simulink model "axi_stream_template"  (R2018a)
settings: Solver=VariableStepAuto  StartTime=0.0  StopTime=300  RelTol=1e-3
libraries: xbsIndex_r4 x18, hdlsllib x5, simulink x1
settings Model: Creator=David Northcote  LastModifiedBy=David Northcote

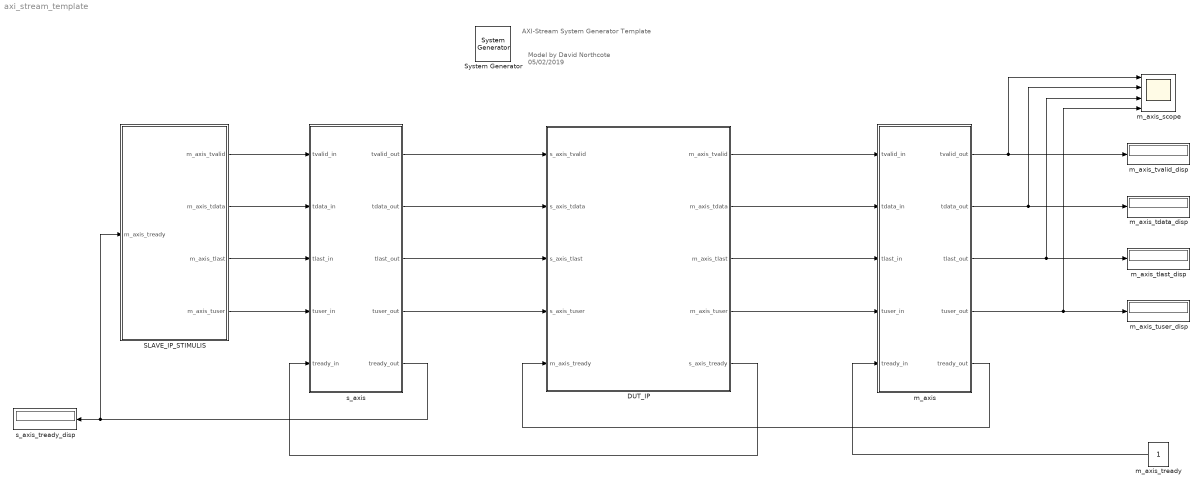
== system axi_stream_template ==
  note: Model by David Northcote
      | 05/02/2019
  note: AXI-Stream System Generator Template
  " System Generator" : xbsIndex_r4/ System Generator  Tag=genX  xilinxfamily=zynq  part=xc7z020  speed=-1  package=clg400  synthesis_tool=Vivado  clock_wrapper=Clock Enables  directory=./netlist  proj_type=Vivado  Synth_file=Vivado Synthesis Defaults  Impl_file=Vivado Implementation Defaults  testbench=off  simulink_period=1  sysclk_period=10  dcm_input_clock_period=10  incr_netlist=off  trim_vbits=Everywhere in SubSystem  dbl_ovrd=According to Block Masks  core_generation=According to Block Masks  run_coregen=off  deprecated_control=off  eval_field=0  block_type=sysgen
  DUT_IP : Subsystem
  SLAVE_IP_STIMULIS : Subsystem
  m_axis : Subsystem
  m_axis_scope : Scope  NumInputPorts=4
  m_axis_tdata_disp : Display
  m_axis_tlast_disp : Display
  m_axis_tready : Constant  VectorParams1D=off  SampleTime=-1
  m_axis_tuser_disp : Display
  m_axis_tvalid_disp : Display
  s_axis : Subsystem
  s_axis_tready_disp : Display
  wires:
  m_axis_tready/1 -> m_axis/5(tready_in)
  s_axis/5(tready_out) -> s_axis_tready_disp/1, SLAVE_IP_STIMULIS/1(m_axis_tready)
  m_axis/1(tvalid_out) -> m_axis_scope/1, m_axis_tvalid_disp/1
  m_axis/3(tlast_out) -> m_axis_scope/3, m_axis_tlast_disp/1
  m_axis/4(tuser_out) -> m_axis_scope/4, m_axis_tuser_disp/1
  m_axis/2(tdata_out) -> m_axis_scope/2, m_axis_tdata_disp/1
  s_axis/1(tvalid_out) -> DUT_IP/1(s_axis_tvalid)
  s_axis/2(tdata_out) -> DUT_IP/2(s_axis_tdata)
  s_axis/3(tlast_out) -> DUT_IP/3(s_axis_tlast)
  s_axis/4(tuser_out) -> DUT_IP/4(s_axis_tuser)
  m_axis/5(tready_out) -> DUT_IP/5(m_axis_tready)
  DUT_IP/5(s_axis_tready) -> s_axis/5(tready_in)
  DUT_IP/1(m_axis_tvalid) -> m_axis/1(tvalid_in)
  DUT_IP/2(m_axis_tdata) -> m_axis/2(tdata_in)
  DUT_IP/3(m_axis_tlast) -> m_axis/3(tlast_in)
  DUT_IP/4(m_axis_tuser) -> m_axis/4(tuser_in)
  SLAVE_IP_STIMULIS/1(m_axis_tvalid) -> s_axis/1(tvalid_in)
  SLAVE_IP_STIMULIS/2(m_axis_tdata) -> s_axis/2(tdata_in)
  SLAVE_IP_STIMULIS/3(m_axis_tlast) -> s_axis/3(tlast_in)
  SLAVE_IP_STIMULIS/4(m_axis_tuser) -> s_axis/4(tuser_in)

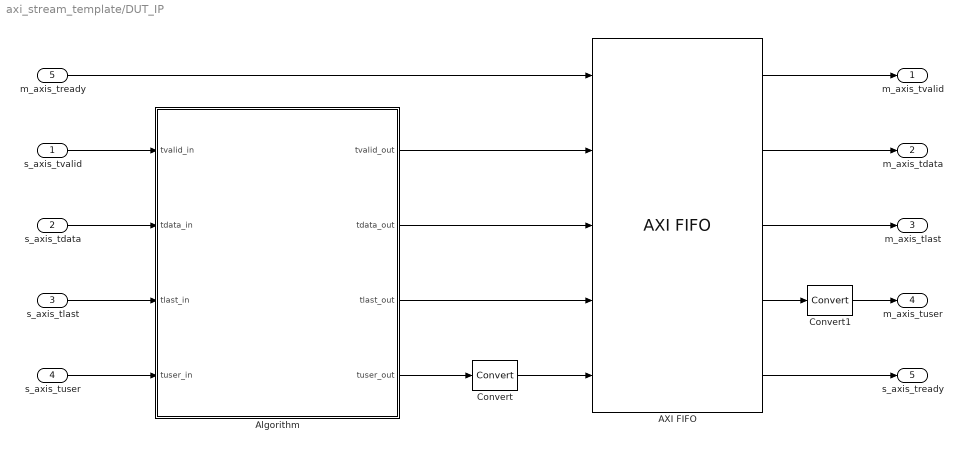
== system axi_stream_template/DUT_IP ==
  s_axis_tvalid : Inport
  s_axis_tdata : Inport  Port=2
  s_axis_tlast : Inport  Port=3
  s_axis_tuser : Inport  Port=4
  m_axis_tready : Inport  Port=5
  AXI FIFO : xbsIndex_r4/AXI FIFO  input_depth_axis=128  actual_fifo_depth_label=130  enable_tdata=on  enable_tdest=off  enable_tstrb=off  enable_tready=on  enable_tid=off  enable_tuser=on  enable_tkeep=off  enable_tlast=on  has_aresetn=off  enable_data_counts_axis=off  fifo_implementation_type_axis=Common Clock Distributed RAM  trim_axipin_name=on  programmable_full_type_axis=Full  full_threshold_assert_value_axis=0  programmable_empty_type_axis=Empty  empty_threshold_assert_value_axis=1022  underflow_flag_axi=0  underflow_sense_axi=Active High  overflow_flag_axi=0  overflow_sense_axi=Active High  block_type=axi_fifo
  Algorithm : Subsystem
  Convert : xbsIndex_r4/Convert  gui_display_data_type=Fixed-point  arith_type=Unsigned  n_bits=1  bin_pt=0  float_type=Single  exp_bits=8  fraction_bits=24  quantization=Truncate  overflow=Wrap  en=off  latency=0  pipeline=off  dbl_ovrd=off  block_type=convert
  Convert1 : xbsIndex_r4/Convert  gui_display_data_type=Boolean  arith_type=Boolean  n_bits=1  bin_pt=0  float_type=Single  exp_bits=8  fraction_bits=24  quantization=Truncate  overflow=Wrap  en=off  latency=0  pipeline=off  dbl_ovrd=off  block_type=convert
  m_axis_tvalid : Outport
  m_axis_tdata : Outport  Port=2
  m_axis_tlast : Outport  Port=3
  m_axis_tuser : Outport  Port=4
  s_axis_tready : Outport  Port=5
  wires:
  AXI FIFO/5 -> s_axis_tready/1
  AXI FIFO/2 -> m_axis_tdata/1
  AXI FIFO/3 -> m_axis_tlast/1
  Algorithm/3(tlast_out) -> AXI FIFO/4
  Algorithm/1(tvalid_out) -> AXI FIFO/2
  AXI FIFO/4 -> Convert1/1
  AXI FIFO/1 -> m_axis_tvalid/1
  Algorithm/2(tdata_out) -> AXI FIFO/3
  Algorithm/4(tuser_out) -> Convert/1
  s_axis_tdata/1 -> Algorithm/2(tdata_in)
  s_axis_tuser/1 -> Algorithm/4(tuser_in)
  s_axis_tvalid/1 -> Algorithm/1(tvalid_in)
  s_axis_tlast/1 -> Algorithm/3(tlast_in)
  m_axis_tready/1 -> AXI FIFO/1
  Convert/1 -> AXI FIFO/5
  Convert1/1 -> m_axis_tuser/1

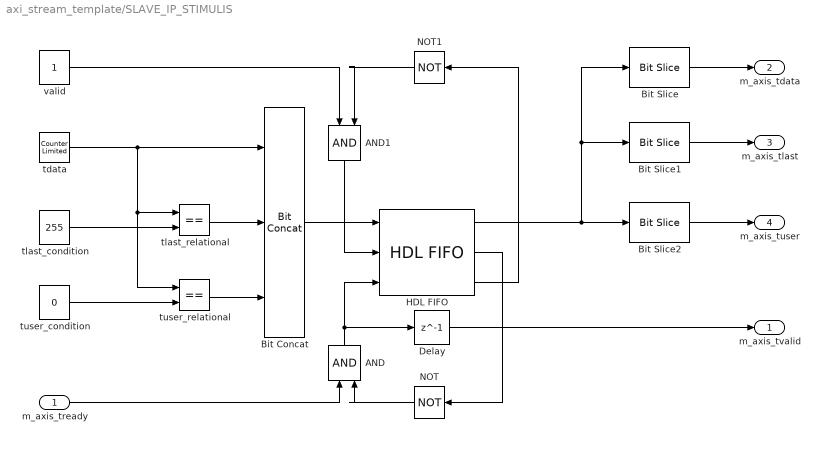
== system axi_stream_template/SLAVE_IP_STIMULIS ==
  m_axis_tready : Inport
  AND : Logic  IconShape=distinctive  AllPortsSameDT=off  OutDataTypeStr=boolean
  AND1 : Logic  IconShape=distinctive  AllPortsSameDT=off  OutDataTypeStr=boolean
  Bit Concat : hdlsllib/Logic and Bit Operations/Bit Concat  numInputs=3
      settings: SourceProductName=HDL Coder  SourceProductBaseCode=HD
  Bit Slice : hdlsllib/Logic and Bit Operations/Bit Slice  lidx=9  ridx=2
  Bit Slice1 : hdlsllib/Logic and Bit Operations/Bit Slice  lidx=1  ridx=1
  Bit Slice2 : hdlsllib/Logic and Bit Operations/Bit Slice  lidx=0  ridx=0
  Delay : Delay  DelayLength=1
  HDL FIFO : hdlsllib/HDL RAMs/HDL FIFO  fifo_size=16  ratio=1  push_msg=Error  pop_msg=Error  show_empty=on  show_full=on  show_num=off
      settings: SourceProductName=HDL Coder  SourceProductBaseCode=HD
  NOT : Logic  Operator=NOT  IconShape=distinctive  AllPortsSameDT=off  OutDataTypeStr=boolean
  NOT1 : Logic  Operator=NOT  IconShape=distinctive  AllPortsSameDT=off  OutDataTypeStr=boolean
  tdata : simulink/Sources/Counter Limited  uplimit=255  tsamp=-1
  tlast_condition : Constant  Value=255  VectorParams1D=off  SampleTime=-1
  tlast_relational : RelationalOperator  Operator===  OutDataTypeStr=boolean  RndMeth=Nearest
  tuser_condition : Constant  Value=0  VectorParams1D=off  SampleTime=-1
  tuser_relational : RelationalOperator  Operator===  OutDataTypeStr=boolean  RndMeth=Nearest
  valid : Constant  VectorParams1D=off
  m_axis_tvalid : Outport
  m_axis_tdata : Outport  Port=2
  m_axis_tlast : Outport  Port=3
  m_axis_tuser : Outport  Port=4
  wires:
  AND/1 -> Delay/1, HDL FIFO/3
  valid/1 -> AND1/1
  NOT/1 -> AND/2
  tlast_condition/1 -> tlast_relational/2
  tlast_relational/1 -> Bit Concat/2
  tdata/1 -> Bit Concat/1, tuser_relational/1, tlast_relational/1
  AND1/1 -> HDL FIFO/2
  tuser_relational/1 -> Bit Concat/3
  HDL FIFO/1 -> Bit Slice2/1, Bit Slice1/1, Bit Slice/1
  Bit Concat/1 -> HDL FIFO/1
  tuser_condition/1 -> tuser_relational/2
  HDL FIFO/2 -> NOT/1
  HDL FIFO/3 -> NOT1/1
  Bit Slice/1 -> m_axis_tdata/1
  m_axis_tready/1 -> AND/1
  Bit Slice2/1 -> m_axis_tuser/1
  Delay/1 -> m_axis_tvalid/1
  Bit Slice1/1 -> m_axis_tlast/1
  NOT1/1 -> AND1/2

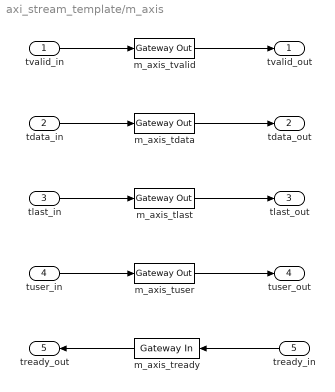
== system axi_stream_template/m_axis ==
  tvalid_in : Inport
  tdata_in : Inport  Port=2
  tlast_in : Inport  Port=3
  tuser_in : Inport  Port=4
  tready_in : Inport  Port=5
  m_axis_tdata : xbsIndex_r4/Gateway Out  inherit_from_input=off  hdl_port=on  rows=1  columns=1  UseAsDAC=off  DACChannel='1'  interface=None  automatic_assignment=on  address_offset=hex2dec('00')  intf_name=''  intf_description=''  timing_constraint=None  locs_specified=off  LOCs={}  io_standard={}  block_type=gatewayout
  m_axis_tlast : xbsIndex_r4/Gateway Out  inherit_from_input=off  hdl_port=on  rows=1  columns=1  UseAsDAC=off  DACChannel='1'  interface=None  automatic_assignment=on  address_offset=hex2dec('00')  intf_name=''  intf_description=''  timing_constraint=None  locs_specified=off  LOCs={}  io_standard={}  block_type=gatewayout
  m_axis_tready : xbsIndex_r4/Gateway In  gui_display_data_type=Boolean  arith_type=Boolean  n_bits=16  bin_pt=14  preci_type=Single  exp_width=8  frac_width=24  rows=1  columns=1  quantization="Round  (unbiased: +/- Inf)"  overflow=Saturate  period=1  UseAsADC=off  ADCChannel='1'  interface=None  automatic_assignment=on  address_offset=hex2dec('00')  intf_name=''  intf_description=''  default_value=0  timing_constraint=None  locs_specified=off  LOCs={}  io_standard={}  inherit_from_input=off  hdl_port=on  dbl_ovrd=off  block_type=gatewayin
  m_axis_tuser : xbsIndex_r4/Gateway Out  inherit_from_input=off  hdl_port=on  rows=1  columns=1  UseAsDAC=off  DACChannel='1'  interface=None  automatic_assignment=on  address_offset=hex2dec('00')  intf_name=''  intf_description=''  timing_constraint=None  locs_specified=off  LOCs={}  io_standard={}  block_type=gatewayout
  m_axis_tvalid : xbsIndex_r4/Gateway Out  inherit_from_input=off  hdl_port=on  rows=1  columns=1  UseAsDAC=off  DACChannel='1'  interface=None  automatic_assignment=on  address_offset=hex2dec('00')  intf_name=''  intf_description=''  timing_constraint=None  locs_specified=off  LOCs={}  io_standard={}  block_type=gatewayout
  tvalid_out : Outport
  tdata_out : Outport  Port=2
  tlast_out : Outport  Port=3
  tuser_out : Outport  Port=4
  tready_out : Outport  Port=5
  wires:
  m_axis_tuser/1 -> tuser_out/1
  tlast_in/1 -> m_axis_tlast/1
  tuser_in/1 -> m_axis_tuser/1
  tvalid_in/1 -> m_axis_tvalid/1
  m_axis_tready/1 -> tready_out/1
  m_axis_tdata/1 -> tdata_out/1
  m_axis_tlast/1 -> tlast_out/1
  tdata_in/1 -> m_axis_tdata/1
  tready_in/1 -> m_axis_tready/1
  m_axis_tvalid/1 -> tvalid_out/1

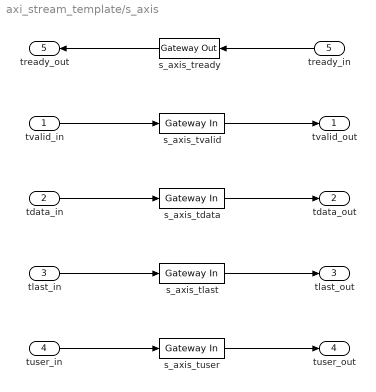
== system axi_stream_template/s_axis ==
  tvalid_in : Inport
  tdata_in : Inport  Port=2
  tlast_in : Inport  Port=3
  tuser_in : Inport  Port=4
  tready_in : Inport  Port=5
  s_axis_tdata : xbsIndex_r4/Gateway In  gui_display_data_type=Fixed-point  arith_type=Unsigned  n_bits=32  bin_pt=0  preci_type=Single  exp_width=8  frac_width=24  rows=1  columns=1  quantization="Round  (unbiased: +/- Inf)"  overflow=Saturate  period=1  UseAsADC=off  ADCChannel='1'  interface=None  automatic_assignment=on  address_offset=hex2dec('00')  intf_name=''  intf_description=''  default_value=0  timing_constraint=None  locs_specified=off  LOCs={}  io_standard={}  inherit_from_input=off  hdl_port=on  dbl_ovrd=off  block_type=gatewayin
  s_axis_tlast : xbsIndex_r4/Gateway In  gui_display_data_type=Boolean  arith_type=Boolean  n_bits=16  bin_pt=14  preci_type=Single  exp_width=8  frac_width=24  rows=1  columns=1  quantization="Round  (unbiased: +/- Inf)"  overflow=Saturate  period=1  UseAsADC=off  ADCChannel='1'  interface=None  automatic_assignment=on  address_offset=hex2dec('00')  intf_name=''  intf_description=''  default_value=0  timing_constraint=None  locs_specified=off  LOCs={}  io_standard={}  inherit_from_input=off  hdl_port=on  dbl_ovrd=off  block_type=gatewayin
  s_axis_tready : xbsIndex_r4/Gateway Out  inherit_from_input=off  hdl_port=on  rows=1  columns=1  UseAsDAC=off  DACChannel='1'  interface=None  automatic_assignment=on  address_offset=hex2dec('00')  intf_name=''  intf_description=''  timing_constraint=None  locs_specified=off  LOCs={}  io_standard={}  block_type=gatewayout
  s_axis_tuser : xbsIndex_r4/Gateway In  gui_display_data_type=Boolean  arith_type=Boolean  n_bits=16  bin_pt=14  preci_type=Single  exp_width=8  frac_width=24  rows=1  columns=1  quantization="Round  (unbiased: +/- Inf)"  overflow=Saturate  period=1  UseAsADC=off  ADCChannel='1'  interface=None  automatic_assignment=on  address_offset=hex2dec('00')  intf_name=''  intf_description=''  default_value=0  timing_constraint=None  locs_specified=off  LOCs={}  io_standard={}  inherit_from_input=off  hdl_port=on  dbl_ovrd=off  block_type=gatewayin
  s_axis_tvalid : xbsIndex_r4/Gateway In  gui_display_data_type=Boolean  arith_type=Boolean  n_bits=16  bin_pt=14  preci_type=Single  exp_width=8  frac_width=24  rows=1  columns=1  quantization="Round  (unbiased: +/- Inf)"  overflow=Saturate  period=1  UseAsADC=off  ADCChannel='1'  interface=None  automatic_assignment=on  address_offset=hex2dec('00')  intf_name=''  intf_description=''  default_value=0  timing_constraint=None  locs_specified=off  LOCs={}  io_standard={}  inherit_from_input=off  hdl_port=on  dbl_ovrd=off  block_type=gatewayin
  tvalid_out : Outport
  tdata_out : Outport  Port=2
  tlast_out : Outport  Port=3
  tuser_out : Outport  Port=4
  tready_out : Outport  Port=5
  wires:
  tready_in/1 -> s_axis_tready/1
  s_axis_tdata/1 -> tdata_out/1
  tdata_in/1 -> s_axis_tdata/1
  s_axis_tready/1 -> tready_out/1
  tlast_in/1 -> s_axis_tlast/1
  tuser_in/1 -> s_axis_tuser/1
  s_axis_tlast/1 -> tlast_out/1
  s_axis_tuser/1 -> tuser_out/1
  tvalid_in/1 -> s_axis_tvalid/1
  s_axis_tvalid/1 -> tvalid_out/1

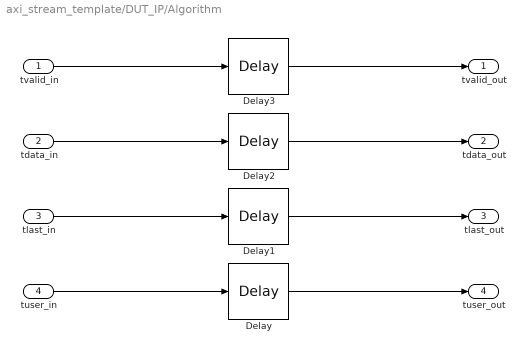
== system axi_stream_template/DUT_IP/Algorithm ==
  tvalid_in : Inport
  tdata_in : Inport  Port=2
  tlast_in : Inport  Port=3
  tuser_in : Inport  Port=4
  Delay{,1..3} (4 alike) : xbsIndex_r4/Delay  rst=off  infoeditControl=Selection of Reset will increase slice count due to use of real FFs and instead of SRLs  en=off  latency=1  reg_retiming=off  dbl_ovrd=off  block_type=delay
  tvalid_out : Outport
  tdata_out : Outport  Port=2
  tlast_out : Outport  Port=3
  tuser_out : Outport  Port=4
  wires:
  Delay/1 -> tuser_out/1
  Delay2/1 -> tdata_out/1
  tvalid_in/1 -> Delay3/1
  tuser_in/1 -> Delay/1
  Delay3/1 -> tvalid_out/1
  Delay1/1 -> tlast_out/1
  tdata_in/1 -> Delay2/1
  tlast_in/1 -> Delay1/1
